simulink model "krzywdalab8_ss_si"  (R2023b)
settings: Solver=VariableStepAuto  StartTime=0.0  StopTime=10.0  RelTol=1e-3
values from neighbouring files (symbols this model uses):
  A = [(-a_1/A1) a_1/A1; a_1/A2 (-a_1 - a_2)/A2]    [feedback_cascade_state.m]    (also in feedback_cascade_transfer_function.m = 2; krzywdalab8.m = [(-a1/A1) a1/A1; a1/A2 (-a1 - a2)/A2])
  B = [1/A1 0; 0 1/A2]    [feedback_cascade_state.m]    (also in krzywdalab8.m)
  C = [1 0; 0 1]    [feedback_cascade_state.m]    (also in krzywdalab8.m)
  D = [0 0; 0 0]    [feedback_cascade_state.m]    (also in krzywdalab8.m)
  dfwe1 = 0.1 * fwe1max    [krzywdalab8.m]
  dfwe2 = 0    [krzywdalab8.m]
  fwe10 = tab_fwe1(it)    [krzywdalab8.m]
  fwe20 = 0.1 * fwe2max    [krzywdalab8.m]
  H0 = [h10 h20]    [krzywdalab8.m]
  T0 = 2    [feedback_cascade_state.m]    (also in feedback_cascade_transfer_function.m; krzywdalab8.m)
settings Model: Creator=igorkrzywda  LastModifiedBy=igorkrzywda

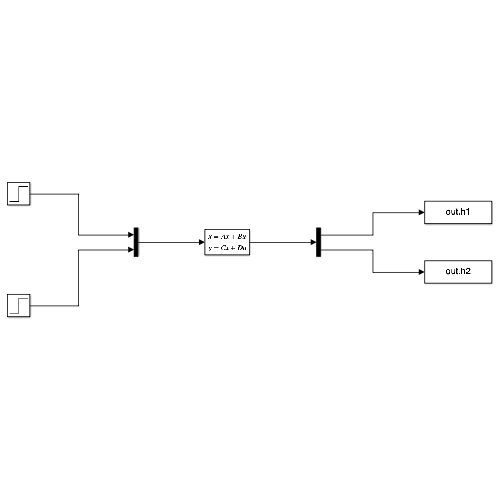
[thumbnail: Simulink's stored preview of the top-level diagram]
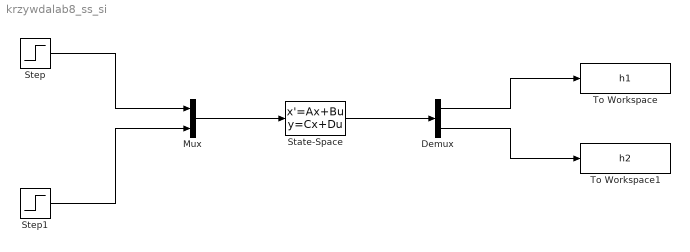
== system krzywdalab8_ss_si ==
  Demux : Demux  Outputs=2
  Mux : Mux  Inputs=2
  State-Space : StateSpace  A=A  B=B  C=C  D=D  InitialCondition=H0
  Step : Step  Time=T0  Before=fwe10  After=fwe10 + dfwe1  SampleTime=0
  Step1 : Step  Time=T0  Before=fwe20  After=fwe20 + dfwe2  SampleTime=0
  To Workspace : ToWorkspace  VariableName=h1  SampleTime=-1
  To Workspace1 : ToWorkspace  VariableName=h2  SampleTime=-1
  wires:
  Mux/1 -> State-Space/1
  State-Space/1 -> Demux/1
  Step/1 -> Mux/1
  Step1/1 -> Mux/2
  Demux/1 -> To Workspace/1
  Demux/2 -> To Workspace1/1
